simulink model "lclowpass_4"  (R2016b)
settings: Solver=ode15s  StartTime=0.0  StopTime=10  RelTol=1e-3
values from neighbouring files (symbols this model uses):
  L = 5    [rlcsolver.m]
  PerT = 0.02    [rlcsolver.m]
  PerV = 30    [rlcsolver.m]
  R = .00192    (= 0.00192)    [rlcsolver.m]
undefined symbols (not defined in the file or in its folder): C
settings Model: Creator=Brian  LastModifiedBy=Brian

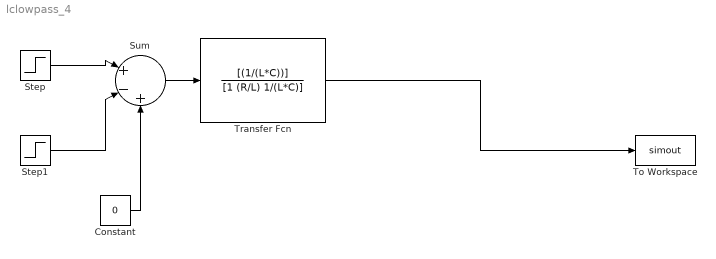
== system lclowpass_4 ==
  Constant : Constant  Value=0
  Step : Step  Time=0  After=PerV  SampleTime=0
  Step1 : Step  Time=PerT  After=PerV  SampleTime=0
  Sum : Sum  Inputs=|+-+
  To Workspace : ToWorkspace  VariableName=simout  SaveFormat=Timeseries  SampleTime=-1
  Transfer Fcn : TransferFcn  Numerator=[(1/(L*C))]  Denominator=[1 (R/L) 1/(L*C)]
  wires:
  Transfer Fcn/1 -> To Workspace/1
  Sum/1 -> Transfer Fcn/1
  Step/1 -> Sum/1
  Step1/1 -> Sum/2
  Constant/1 -> Sum/3
